simulink model "Sim_Delay"  (R2021a)
settings: Solver=FixedStepAuto  StartTime=0.0  StopTime=tf  FixedStep=Ts  RelTol=1e-3
undefined symbols (not defined in the file): Noise, Ts, TWindow
libraries: simulink x1
settings Model: Creator=perruquetti  LastModifiedBy=perruquetti

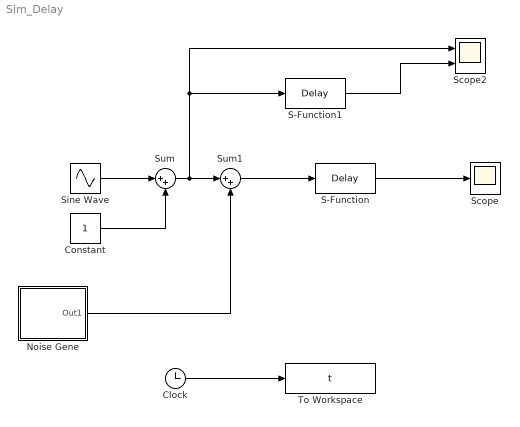
== system Sim_Delay ==
  Clock : Clock
  Constant : Constant
  Noise Gene : Subsystem
  S-Function : S-Function  FunctionName=Delay  Parameters=Ts,TWindow  SFunctionDeploymentMode=off  EnableBusSupport=off
  S-Function1 : S-Function  FunctionName=Delay  Parameters=Ts,TWindow  SFunctionDeploymentMode=off  EnableBusSupport=off
  Scope : Scope
  Scope2 : Scope  NumInputPorts=2
  Sine Wave : Sin  Frequency=10  SampleTime=0
  Sum : Sum  Inputs=|++
  Sum1 : Sum  Inputs=|++
  To Workspace : ToWorkspace  VariableName=t  SampleTime=-1
  wires:
  Constant/1 -> Sum/2
  Sine Wave/1 -> Sum/1
  Clock/1 -> To Workspace/1
  Sum1/1 -> S-Function/1
  Sum/1 -> S-Function1/1, Scope2/1, Sum1/1
  Noise Gene/1(Out1) -> Sum1/2
  S-Function1/1 -> Scope2/2
  S-Function/1 -> Scope/1

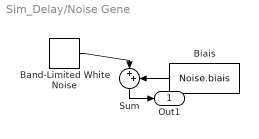
== system Sim_Delay/Noise Gene ==
  Band-Limited White Noise : simulink/Sources/Band-Limited White Noise  Cov=Noise.power  Ts=Noise.sampling  seed=Noise.seed
  Biais : Constant  Value=Noise.biais
  Sum : Sum  Inputs=|++
  Out1 : Outport
  wires:
  Sum/1 -> Out1/1
  Biais/1 -> Sum/2
  Band-Limited White Noise/1 -> Sum/1
